simulink model "block2_simulink"  (R2025a)
settings: Solver=ode23tb  StartTime=0.0  StopTime=9  RelTol=1e-3
values from neighbouring files (symbols this model uses):
  C = 1.05 * C_min    (= 4.1015625e-05)    [Block2.m]
  G = 1.25/vC_nom^2    (= 0.0048828125)    [Block2.m]
  I0_nom = P_nom/vC_nom    (= 6.25)    [Block2.m]
  iL_nom = P_nom/(n*V0)    (= 8.77192982456)    [Block2.m]
  Jac_A_lin = double(subs(Jac_A, {vC, iL, u}, {vC_nom, iL_bar, u_bar}))    [Block2.m]
  Jac_B_lin = double(subs(Jac_B, {vC, iL, u}, {vC_nom, iL_bar, u_bar}))    [Block2.m]
  Ki = 10    [Block2.m]
  Ki_c = 200    [Block2.m]
  Kp = 0.1    [Block2.m]
  Kp_c = 500    [Block2.m]
  L = 1.05 * L_min    (= 0.0001008)    [Block2.m]
  R = 3.75/iL_nom^2    (= 0.048735)    [Block2.m]
  V0 = 12    [Block2.m]
  vC_nom = 16    [Block2.m]
libraries: SignalEditorBlockLib x1
settings Model: Creator=arntzen  LastModifiedBy=Markus

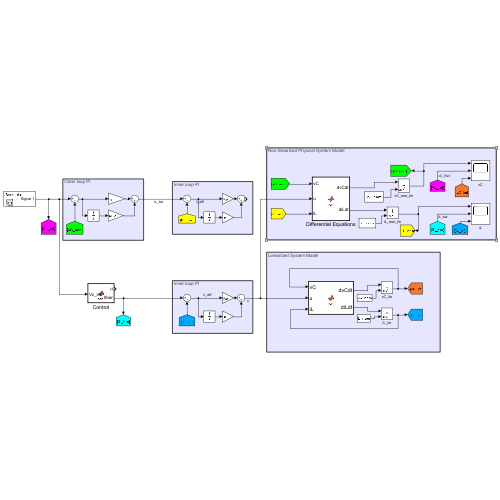
[thumbnail: Simulink's stored preview of the top-level diagram]
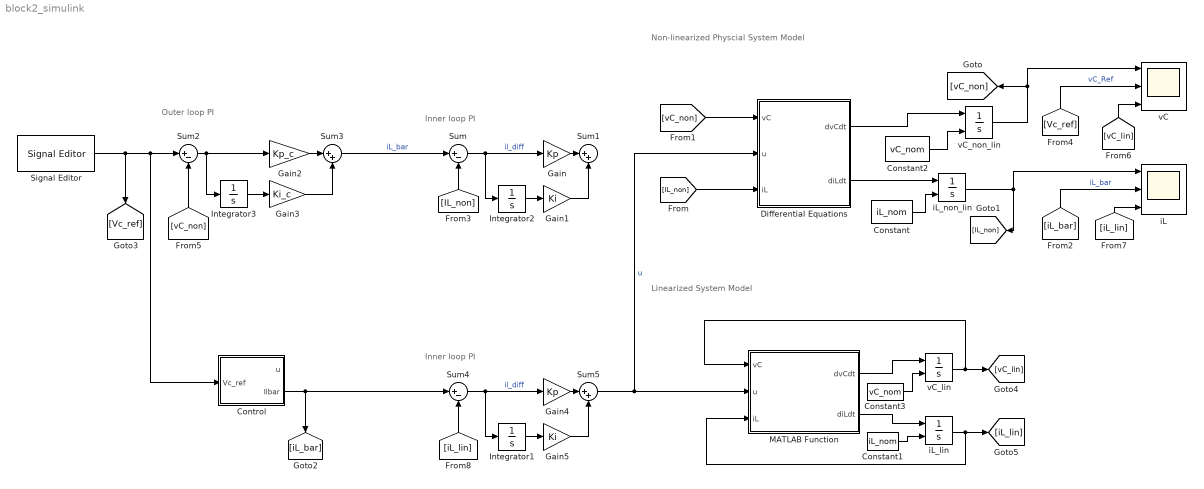
== system block2_simulink ==
  note: Linearized System Model
  note: Inner loop PI
  note: Outer loop PI
  note: Non-linearized Physcial System Model
  note: Inner loop PI
  Constant : Constant  Value=iL_nom
  Constant1 : Constant  Value=iL_nom
  Constant2 : Constant  Value=vC_nom
  Constant3 : Constant  Value=vC_nom
  Control : MATLAB Function  TreatAsAtomicUnit=on
  Differential Equations : MATLAB Function  TreatAsAtomicUnit=on
  Gain : Gain  Gain=Kp
  Gain1 : Gain  Gain=Ki
  Gain2 : Gain  Gain=Kp_c
  Gain3 : Gain  Gain=Ki_c
  Gain4 : Gain  Gain=Kp
  Gain5 : Gain  Gain=Ki
  Integrator1 : Integrator
  Integrator2 : Integrator
  Integrator3 : Integrator
  MATLAB Function : MATLAB Function  TreatAsAtomicUnit=on
  Signal Editor : SignalEditorBlockLib/Signal Editor  FileName=Block_2_signaleditor.mat  ActiveScenario=Scenario  ActiveSignal=Signal 1  IsBus=off  OutputBusObjectStr=Bus: BusObject  SampleTime=0  ZeroCross=off  OutputAfterFinalValue=Setting to zero  Unit=inherit  PreserveSignalName=on  ApplySigPropsToAllScenarios=on  ApplySigPropsToAllSignals=off  SignalPropertySource=Dialog parameters
  Sum : Sum  Inputs=|+-
  Sum1 : Sum  Inputs=|++
  Sum2 : Sum  Inputs=|+-
  Sum3 : Sum  Inputs=|++
  Sum4 : Sum  Inputs=|+-
  Sum5 : Sum  Inputs=|++
  iL : Scope  NumInputPorts=3
      settings: ActiveDisplayYMinimum=8.2133862835336  ActiveDisplayYMaximum=8.4809768431811126
  iL_lin : Integrator  InitialConditionSource=external
  iL_non_lin : Integrator  InitialConditionSource=external
  vC : Scope  NumInputPorts=3
      settings: ActiveDisplayYMinimum=6.3448607643623163  ActiveDisplayYMaximum=22.896253120739157
  vC_lin : Integrator  InitialConditionSource=external
  vC_non_lin : Integrator  InitialConditionSource=external
  wires:
  Differential Equations/1(dvCdt) -> vC_non_lin/1
  [IL_non] -> Differential Equations/3(iL)
  [vC_non] -> Differential Equations/1(vC)
  Constant2/1 -> vC_non_lin/2
  vC_non_lin/1 -> [vC_non], vC/1
  Differential Equations/2(diLdt) -> iL_non_lin/1
  iL_non_lin/1 -> [IL_non], iL/1
  Constant/1 -> iL_non_lin/2
  Sum/1 -> Integrator2/1, Gain/1  "il_diff"
  [IL_non] -> Sum/2
  Gain/1 -> Sum1/1
  Gain1/1 -> Sum1/2
  Sum2/1 -> Gain2/1, Integrator3/1
  Signal Editor/1 -> Control/1(Vc_ref), Sum2/1, [Vc_ref]
  [vC_non] -> Sum2/2
  Integrator3/1 -> Gain3/1
  Gain3/1 -> Sum3/2
  Gain2/1 -> Sum3/1
  Sum3/1 -> Sum/1  "iL_bar"
  Integrator2/1 -> Gain1/1
  MATLAB Function/1(dvCdt) -> vC_lin/1
  MATLAB Function/2(diLdt) -> iL_lin/1
  vC_lin/1 -> MATLAB Function/1(vC), [vC_lin]
  iL_lin/1 -> [iL_lin], MATLAB Function/3(iL)
  [iL_bar] -> iL/2  "iL_bar"
  [Vc_ref] -> vC/2  "vC_Ref"
  Constant3/1 -> vC_lin/2
  Constant1/1 -> iL_lin/2
  [vC_lin] -> vC/3
  [iL_lin] -> iL/3
  Control/2(Ilbar) -> [iL_bar], Sum4/1
  Gain5/1 -> Sum5/2
  Gain4/1 -> Sum5/1
  Sum4/1 -> Integrator1/1, Gain4/1  "il_diff"
  Integrator1/1 -> Gain5/1
  [iL_lin] -> Sum4/2
  Sum5/1 -> Differential Equations/2(u), MATLAB Function/2(u)  "u"

== matlab function block2_simulink/Control ==
  data: u output; V0 parameter; R parameter; G parameter; I0_nom parameter; Vc_ref input; Ilbar output
function [u, Ilbar] = fcn(V0, R, G, I0_nom, Vc_ref)

Ilbar = (V0 - sqrt(V0^2 - 4*R*(G*Vc_ref^2 + I0_nom*Vc_ref))) / (2*R);
u = 1 - (G*Vc_ref + I0_nom) / Ilbar;

== matlab function block2_simulink/Differential Equations ==
  data: R parameter; G parameter; V0 parameter; dvCdt output; I0_nom parameter; diLdt output; vC input; u input; iL input; L parameter; C parameter
%function [dILdt, dVcdt] = fcn(R, C, L, V0, G, I0_nom, Vc_nom)
function [dvCdt, diLdt] = fcn(R, G, V0, I0_nom, vC, u, iL, L, C)

dvCdt = -G/C*vC + (1-u)/C*iL - I0_nom/C
diLdt = -R/L*iL - (1-u)/L*vC + V0/L

== matlab function block2_simulink/MATLAB Function ==
  data: vC input; u input; iL input; dvCdt output; Jac_A_lin parameter; Jac_B_lin parameter; E parameter; diLdt output
function [dvCdt, diLdt]  = fcn(vC, u, iL, Jac_A_lin, Jac_B_lin, E)

x = [iL
     vC]

dxdt = Jac_A_lin * x + Jac_B_lin * u + E;

diLdt = dxdt(1);
dvCdt = dxdt(2);
